simulink model "spwm"  (R2022a)
settings: Solver=ode4  StartTime=0.0  StopTime=0.5  FixedStep=1e-5  RelTol=1e-3
values from neighbouring files (symbols this model uses):
  f = 50    [untitled.m]
  V_input = 550    [untitled.m]
libraries: spsIGBTDiodeLib x6, spsDCVoltageSourceLib x1, spsGroundLib x1, simulink x1, spsThreePhaseSeriesRLCBranchLib x1, spsThreePhaseVIMeasurementLib x1, spspowerguiLib x1
settings Model: Creator=hp  LastModifiedBy=hp

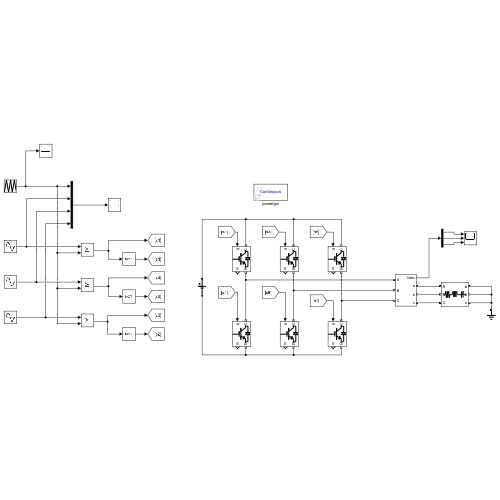
[thumbnail: Simulink's stored preview of the top-level diagram]
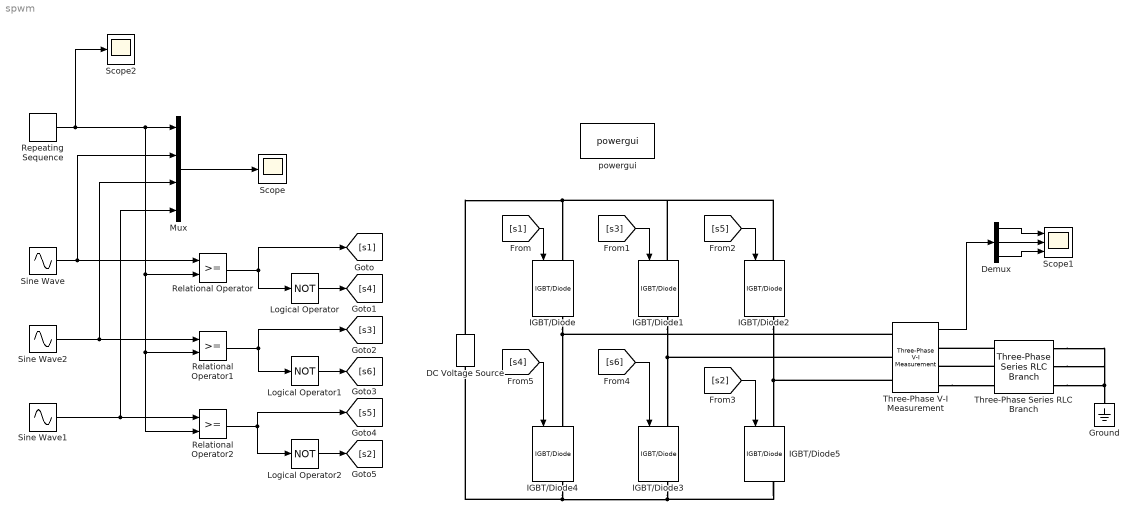
== system spwm ==
  DC Voltage Source : spsDCVoltageSourceLib/DC Voltage Source  Amplitude=V_input  Measurements=None
  Demux : Demux  Outputs=3
  Ground : spsGroundLib/Ground  LConnTagsString=a
  IGBT/Diode{,1..5} (6 alike) : spsIGBTDiodeLib/IGBT//Diode  Ron=1e-3  Rs=1e5  Cs=inf  Measurements=on
  Logical Operator : Logic  Operator=NOT  AllPortsSameDT=off  OutDataTypeStr=boolean
  Logical Operator1 : Logic  Operator=NOT  AllPortsSameDT=off  OutDataTypeStr=boolean
  Logical Operator2 : Logic  Operator=NOT  AllPortsSameDT=off  OutDataTypeStr=boolean
  Mux : Mux
  Relational Operator : RelationalOperator  OutDataTypeStr=boolean  RndMeth=Simplest  InputSameDT=off
  Relational Operator1 : RelationalOperator  OutDataTypeStr=boolean  RndMeth=Simplest  InputSameDT=off
  Relational Operator2 : RelationalOperator  OutDataTypeStr=boolean  RndMeth=Simplest  InputSameDT=off
  Repeating Sequence : simulink/Sources/Repeating Sequence  rep_seq_t=[0 5e-4 1e-3]  rep_seq_y=[-250 250 -250]
  Scope : Scope
  Scope1 : Scope  NumInputPorts=3
  Scope2 : Scope
  Sine Wave : Sin  Amplitude=256  Frequency=2*pi*f  SampleTime=0
  Sine Wave1 : Sin  Amplitude=256  Frequency=2*pi*f  Phase=2*pi/3  SampleTime=0
  Sine Wave2 : Sin  Amplitude=256  Frequency=2*pi*f  Phase=-2*pi/3  SampleTime=0
  Three-Phase Series RLC Branch : spsThreePhaseSeriesRLCBranchLib/Three-Phase Series RLC Branch  LConnTagsString=A|B|C  RConnTagsString=A|B|C  BranchType=RLC  Resistance=10  Inductance=1e-3  Capacitance=0  Measurements=None
  Three-Phase V-I Measurement : spsThreePhaseVIMeasurementLib/Three-Phase V-I Measurement  VoltageMeasurement=phase-to-ground  SetLabelV=off  LabelV=Vabc  Vpu=off  VpuLL=off  CurrentMeasurement=no  SetLabelI=off  LabelI=Iabc  Ipu=off  Pbase=100e6  Vbase=500e3  OutputType=Complex  PhasorSimulation=off  PSBequivalent=0
  powergui : spspowerguiLib/powergui  Priority=1  SimulationMode=Continuous  SampleTime=50e-6  frequency=60  Iterations=50  frequencyindice=0  Pbase=100e6  ErrMax=1e-4  UnitsV=kV  UnitsW=MW  buscounter=0  FunctionMessages=off  echomessages=off  EnableUseOfTLC=off  CurrentSourceSwitches=off  DisableSnubberDevices=off  DisableRonSwitches=off  DisableVfSwitches=off  DisplayEquations=off  AutomaticDiscreteSolvers=off  SolverType=Tustin/Backward Euler (TBE)  Interpol=off  ExternalGateDelay=off  methode=off  Ts=100  x0status=blocks  SPID=on  SwTol=0  HookPort=off  NonlinearTolerance=1e-4  nMaxIteration=100  ContinueOnMaxIteration=off  RestoreLinks=warning  ResistiveCurrentMeasurement=off  Frange=[0:2:500]  Ylog=off  Xlog=on  ShowGrid=off  save=off  variable=ZData  structure=0  ZoomFFT=off  StartTime=0.0  cycles=1  DisplayStyle=1  fundamental=60  FreqAxis=off  MaxFrequency=1000  frequencyindicesteady=1  RmsSteady=1  display=off
  wires:
  Sine Wave/1 -> Relational Operator/1, Mux/2
  Sine Wave2/1 -> Relational Operator1/1, Mux/3
  Mux/1 -> Scope/1
  Repeating Sequence/1 -> Scope2/1, Relational Operator2/2, Relational Operator1/2, Relational Operator/2, Mux/1
  Sine Wave1/1 -> Mux/4, Relational Operator2/1
  Logical Operator/1 -> [s4]
  Relational Operator/1 -> [s1], Logical Operator/1
  Logical Operator1/1 -> [s6]
  Relational Operator1/1 -> Logical Operator1/1, [s3]
  Logical Operator2/1 -> [s2]
  Relational Operator2/1 -> Logical Operator2/1, [s5]
  [s1] -> IGBT/Diode/1
  [s3] -> IGBT/Diode1/1
  [s5] -> IGBT/Diode2/1
  [s2] -> IGBT/Diode5/1
  [s6] -> IGBT/Diode3/1
  [s4] -> IGBT/Diode4/1
  Demux/2 -> Scope1/2
  Demux/1 -> Scope1/1
  Demux/3 -> Scope1/3
  Three-Phase V-I Measurement/1 -> Demux/1
  connections:
  IGBT/Diode/RConn1 -- Three-Phase V-I Measurement/LConn1 -- IGBT/Diode4/LConn1
  DC Voltage Source/RConn1 -- IGBT/Diode/LConn1 -- IGBT/Diode1/LConn1 -- IGBT/Diode2/LConn1
  IGBT/Diode4/RConn1 -- IGBT/Diode5/RConn1 -- IGBT/Diode3/RConn1 -- DC Voltage Source/LConn1
  Three-Phase Series RLC Branch/LConn1 -- Three-Phase V-I Measurement/RConn1
  Three-Phase Series RLC Branch/LConn2 -- Three-Phase V-I Measurement/RConn2
  Three-Phase V-I Measurement/RConn3 -- Three-Phase Series RLC Branch/LConn3
  Three-Phase Series RLC Branch/RConn3 -- Three-Phase Series RLC Branch/RConn1 -- Three-Phase Series RLC Branch/RConn2 -- Ground/LConn1
  IGBT/Diode2/RConn1 -- Three-Phase V-I Measurement/LConn3 -- IGBT/Diode5/LConn1
  IGBT/Diode1/RConn1 -- Three-Phase V-I Measurement/LConn2 -- IGBT/Diode3/LConn1
